simulink model "TAULab11"  (R2014b)
settings: Solver=ode45  StartTime=0.0  StopTime=50  RelTol=1e-3
libraries: simulink x2
settings Model: Creator=kiril_000  LastModifiedBy=kiril_000

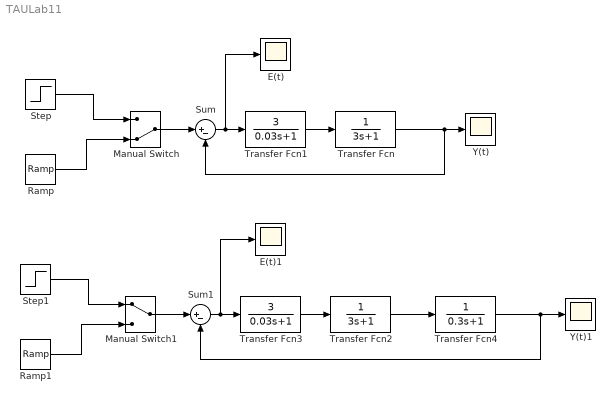
== system TAULab11 ==
  E(t) : Scope
  E(t)1 : Scope
      settings: SaveName=ScopeData2
  Manual Switch : ManualSwitch  CurrentSetting=0
  Manual Switch1 : ManualSwitch
  Ramp : simulink/Sources/Ramp  slope=1  start=0  X0=0
  Ramp1 : simulink/Sources/Ramp  slope=1  start=0  X0=0
  Step : Step  Time=0  SampleTime=0
  Step1 : Step  Time=0  SampleTime=0
  Sum : Sum  Inputs=|+-
  Sum1 : Sum  Inputs=|+-
  Transfer Fcn : TransferFcn  Denominator=[3 1]
  Transfer Fcn1 : TransferFcn  Numerator=[3]  Denominator=[0.03 1]
  Transfer Fcn2 : TransferFcn  Denominator=[3 1]
  Transfer Fcn3 : TransferFcn  Numerator=[3]  Denominator=[0.03 1]
  Transfer Fcn4 : TransferFcn  Denominator=[0.3 1]
  Y(t) : Scope
  Y(t)1 : Scope
      settings: TimeRange=50  YMin=-1.159949421134341e-63  YMax=40  SaveName=ScopeData3
  wires:
  Step/1 -> Manual Switch/1
  Ramp/1 -> Manual Switch/2
  Manual Switch/1 -> Sum/1
  Sum/1 -> E(t)/1, Transfer Fcn1/1
  Transfer Fcn1/1 -> Transfer Fcn/1
  Transfer Fcn/1 -> Sum/2, Y(t)/1
  Step1/1 -> Manual Switch1/1
  Ramp1/1 -> Manual Switch1/2
  Manual Switch1/1 -> Sum1/1
  Sum1/1 -> Transfer Fcn3/1, E(t)1/1
  Transfer Fcn3/1 -> Transfer Fcn2/1
  Transfer Fcn2/1 -> Transfer Fcn4/1
  Transfer Fcn4/1 -> Y(t)1/1, Sum1/2
